simulink model "model"  (R2023a)
settings: Solver=VariableStepAuto  StartTime=0.0  StopTime=50  RelTol=1e-6
values from neighbouring files (symbols this model uses):
  ParSt = MyObject    [main.m]
settings Model: Creator=User  LastModifiedBy=User

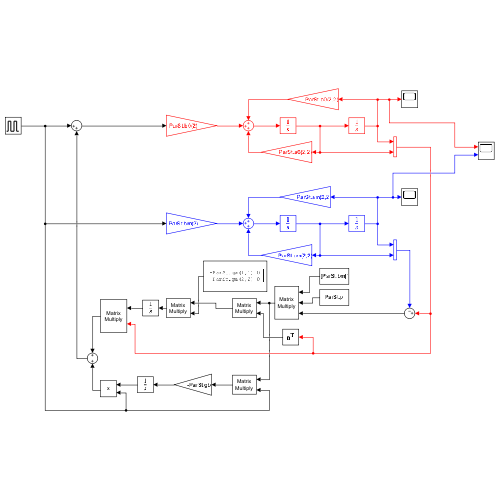
[thumbnail: Simulink's stored preview of the top-level diagram]
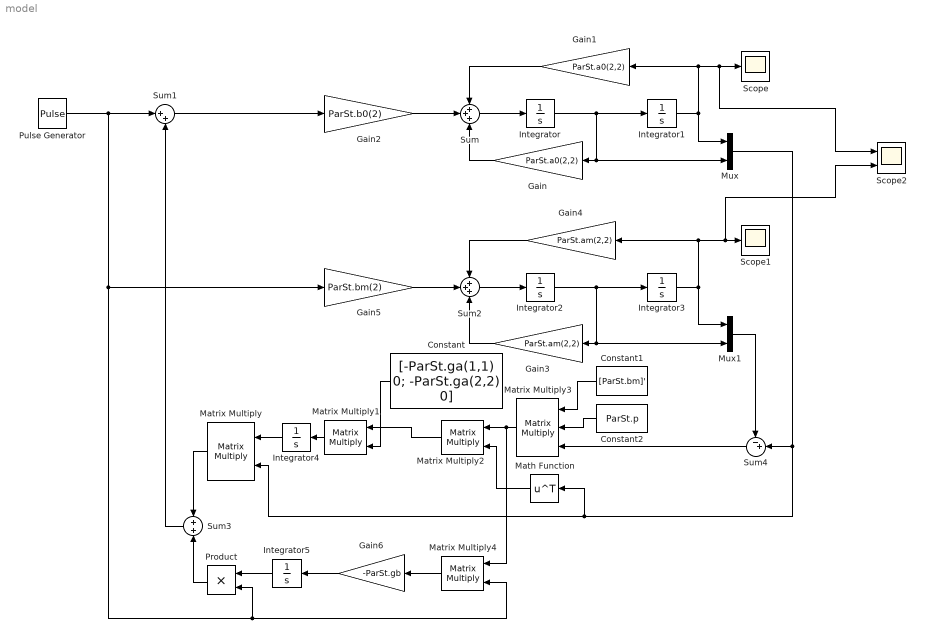
== system model ==
  Constant : Constant  Value=[-ParSt.ga(1,1) 0; -ParSt.ga(2,2) 0]  VectorParams1D=off
  Constant1 : Constant  Value=[ParSt.bm]'  VectorParams1D=off
  Constant2 : Constant  Value=ParSt.p  VectorParams1D=off
  Gain : Gain  Gain=ParSt.a0(2,2)
  Gain1 : Gain  Gain=ParSt.a0(2,2)
  Gain2 : Gain  Gain=ParSt.b0(2)
  Gain3 : Gain  Gain=ParSt.am(2,2)
  Gain4 : Gain  Gain=ParSt.am(2,2)
  Gain5 : Gain  Gain=ParSt.bm(2)
  Gain6 : Gain  Gain=-ParSt.gb
  Integrator{,1..5} (6 alike) : Integrator
  Math Function : Math  Operator=transpose
  Matrix Multiply{,1..2,4} (4 alike) : Product  Multiplication=Matrix(*)
  Matrix Multiply3 : Product  Inputs=3  Multiplication=Matrix(*)
  Mux : Mux  Inputs=2
  Mux1 : Mux  Inputs=2
  Product : Product
  Pulse Generator : DiscretePulseGenerator  PulseType=Time based  Period=20  PulseWidth=50
  Scope : Scope
  Scope1 : Scope
  Scope2 : Scope  NumInputPorts=2
  Sum : Sum  Inputs=+++
  Sum1 : Sum  Inputs=|++
  Sum2 : Sum  Inputs=+++
  Sum3 : Sum
  Sum4 : Sum  Inputs=-+|
  wires:
  Integrator/1 -> Mux/2, Gain/1, Integrator1/1
  Sum/1 -> Integrator/1
  Gain/1 -> Sum/3
  Gain1/1 -> Sum/1
  Integrator1/1 -> Scope2/1, Scope/1, Gain1/1, Mux/1
  Gain2/1 -> Sum/2
  Sum1/1 -> Gain2/1
  Integrator2/1 -> Mux1/2, Gain3/1, Integrator3/1
  Gain3/1 -> Sum2/3
  Gain4/1 -> Sum2/1
  Gain5/1 -> Sum2/2
  Integrator3/1 -> Scope2/2, Scope1/1, Gain4/1, Mux1/1
  Sum2/1 -> Integrator2/1
  Pulse Generator/1 -> Matrix Multiply4/2, Product/2, Gain5/1, Sum1/1
  Mux/1 -> Sum4/2, Math Function/1, Matrix Multiply/2
  Integrator4/1 -> Matrix Multiply/1
  Matrix Multiply1/1 -> Integrator4/1
  Matrix Multiply/1 -> Sum3/1
  Product/1 -> Sum3/2
  Sum3/1 -> Sum1/2
  Matrix Multiply3/1 -> Matrix Multiply4/1, Matrix Multiply2/1
  Math Function/1 -> Matrix Multiply2/2
  Constant1/1 -> Matrix Multiply3/1
  Constant2/1 -> Matrix Multiply3/2
  Sum4/1 -> Matrix Multiply3/3
  Mux1/1 -> Sum4/1
  Integrator5/1 -> Product/1
  Gain6/1 -> Integrator5/1
  Matrix Multiply4/1 -> Gain6/1
  Constant/1 -> Matrix Multiply1/2
  Matrix Multiply2/1 -> Matrix Multiply1/1
